simulink library "Wall_basic"  (R2018b)
settings: Solver=ode45  StartTime=0.0  StopTime=10.0  RelTol=1e-3  EnableMultiTasking=on
settings Model: Creator=drhf  LastModifiedBy=P41573
settings DataIOCC: LimitDataPoints=on  SaveFormat=Array  SignalLoggingSaveFormat=ModelDataLogs
settings OptimizationCC: ExpressionDepthLimit=2147483647  LifeSpan=inf
settings DebuggingCC: UnderspecifiedInitializationDetection=Classic  MergeDetectMultiDrivingBlocksExec=none  SolverPrmCheckMsg=warning  FcnCallInpInsideContextMsg=warning  StateNameClashWarn=warning  SFUnexpectedBacktrackingDiag=warning  SFNoUnconditionalDefaultTransitionDiag=warning  SFExecutionAtInitializationDiag=none
settings HardwareCC: ProdBitPerPointer=32  ProdBitPerSizeT=32  ProdBitPerPtrDiffT=32  ProdLargestAtomicFloat=None  ProdIntDivRoundTo=Undefined  ProdEndianess=Unspecified  ProdWordSize=32  ProdHWDeviceType=32-bit Generic
settings ModelReferenceCC: PropagateSignalLabelsOutOfModel=off
settings SFSimCC: SimUseLocalCustomCode=off
settings RTWCC: RTWUseLocalCustomCode=off
settings CodeAppCC: StateflowObjectComments=on
settings GRTTargetCC: TargetLangStandard=C89/C90 (ANSI)  GeneratePreprocessorConditionals=Disable all  CombineOutputUpdateFcns=off  GRTInterface=on
settings ConfigComp: CovMetricSettings=dw  CovHtmlReporting=on  CovSaveCumulativeToWorkspaceVar=on  CovSaveSingleToWorkspaceVar=on  CovExternalEMLEnable=off

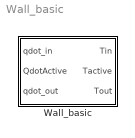
== system Wall_basic ==
  Wall_basic : Subsystem  mask(Wall basic){tau=3600, t0=20, d=[0.1 0.1 0.1], dactive=-1, cond=[1 2 1], cwall=[800 1000 800], rho=[2000 2700 2000]}
      mask prompts: tau "Time constant in s"; t0 "Initial temperature in °C"; d "Thickness of layers in m"; dactive "Depth of active layer(s) in m"; cond "Conductivity of layer material in W/m/K"; cwall "Capacity of layer material in J/kg/K"; rho "Density of layer material in kg/m³"
      mask help: Basic model of a wall using a multilayer Beuken model.
      mask Help: web(fullfile(path_carnot('help'),'Wall_basic.html'),'-helpbrowser')

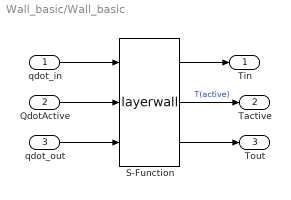
== system Wall_basic/Wall_basic ==
  qdot_in : Inport
  QdotActive : Inport  Port=2
  qdot_out : Inport  Port=3
  S-Function : S-Function  FunctionName=layerwall  Parameters=tau, t0, d, cond, cwall, rho, dactive  SFunctionDeploymentMode=off  EnableBusSupport=off
  Tin : Outport
  Tactive : Outport  Port=2
  Tout : Outport  Port=3
  wires:
  S-Function/3 -> Tout/1
  qdot_out/1 -> S-Function/3
  S-Function/2 -> Tactive/1  "T(active)"
  QdotActive/1 -> S-Function/2
  S-Function/1 -> Tin/1
  qdot_in/1 -> S-Function/1
